simulink model "section4_simulation_editedbyzym"  (R2023b)
settings: Solver=FixedStepAuto  StartTime=0.0  StopTime=620  FixedStep=0.001  RelTol=1e-3
(part 2 of 2)

== matlab function section4_simulation_editedbyzym/droux ==
  data: krou input; y output; rou0 input; rou00 input; t input
function y = fcn(krou,rou0,rou00,t)
u=-krou*(rou0-rou00)*exp(-krou*t);
y = u;

== matlab function section4_simulation_editedbyzym/drouy1 ==
  data: krou input; y output; rou0 input; rou00 input; t input
function y = fcn(krou,rou0,rou00,t)
u=-krou*(rou0-rou00)*exp(-krou*t);
y = u;

== matlab function section4_simulation_editedbyzym/rouy1 ==
  data: rou0 input; y output; rou00 input; krou input; t input
function y = fcn(rou0,rou00,krou,t)
u=(rou0-rou00)*exp(-krou*t)+rou00;
y = u;

== matlab function section4_simulation_editedbyzym/MATLAB Function12 ==
  data: tauiL input; tauiR input; r input; J input; m input; dv1 output; domg1 output; l input
function [dv1,domg1] = fcn(tauiL,tauiR,r,J,m,l)

dv1=(tauiL+tauiR)/(m*r);

domg1=l*(tauiR-tauiL)/(J*r);

== matlab function section4_simulation_editedbyzym/MATLAB Function18 ==
  data: rphiL2 input; y output; thetaL input; theta2 input
function y = fcn(rphiL2,thetaL,theta2)
u=rphiL2+thetaL-theta2-pi/3;
y = u;

== matlab function section4_simulation_editedbyzym/MATLAB Function30 ==
  data: JIL output; JI1 output; JI2 output; JI3 output; x1 input; y1 input; x2 input; y2 input; x3 input; y3 input; xL input; yL input; yil output; sanyi output; yier output; saner output; erl output
function [JIL,JI1,JI2, JI3,yil,sanyi,yier,saner,erl]= fcn(x1,y1,x2,y2,x3,y3,xL,yL)
yil=sqrt((x1-xL)^2+(y1-yL)^2);
erl=sqrt((x2-xL)^2+(y2-yL)^2);
yier=sqrt((x2-x1)^2+(y2-y1)^2);
sanyi=sqrt((x3-x1)^2+(y3-y1)^2);
saner=sqrt((x3-x2)^2+(y3-y2)^2);
sanl=sqrt((x3-xL)^2+(y3-yL)^2);
JL=((yil)^2+(erl)^2-(yier)^2)/(2*yil*erl);
J1=((yil)^2+(sanyi)^2-(sanl)^2)/(2*yil*sanyi);
J2=((erl)^2+(saner)^2-(sanl)^2)/(2*erl*saner);
J3=((sanyi)^2+(saner)^2-(yier)^2)/(2*sanyi*saner);
JIL = acos(JL);
JI1 = acos(J1);
JI2 = acos(J2);
JI3 = acos(J3);

== matlab function section4_simulation_editedbyzym/phiL1 ==
  data: arfji output; xj input; phiji output; xi input; yj input; yi input; thetai input; thetaj input
function [arfji,phiji] = fcn(xj,xi,yj,yi,thetai,thetaj)
xji=cos(thetai)*(xj-xi)+sin(thetai)*(yj-yi);
yji=-sin(thetai)*(xj-xi)+cos(thetai)*(yj-yi);
arfji=atan(yji/xji);
phiji=arfji+thetai-thetaj;

== matlab function section4_simulation_editedbyzym/MATLAB Function1 ==
  data: aa input; tauiL output; bb input; cc input; dd input; uid input; uip input
function tauiL = fcn(aa,bb,cc,dd,uid,uip)

% if aa/bb-cc/dd<0.05 && aa/bb-cc/dd>-0.05
%     tauiL=1\(uid/bb-uip/dd);
% 
% 
% else 
tauiL=(aa/bb-cc/dd)\(uid/bb-uip/dd);
% end

== matlab function section4_simulation_editedbyzym/MATLAB Function2 ==
  data: aa input; tauiR output; bb input; cc input; dd input; uid input; uip input
function tauiR = fcn(aa,bb,cc,dd,uid,uip)

% if aa/bb-cc/dd<0.05 && aa/bb-cc/dd>-0.05
%     tauiR=1\(uid/aa-uip/cc);
% 
% else
tauiR=(bb/aa-dd/cc)\(uid/aa-uip/cc);
% end

== matlab function section4_simulation_editedbyzym/MATLAB Function9 ==
  data: gamma_id input; y output; sigma_id input; Didm_hat input; delta_id input
function y = fcn(gamma_id,sigma_id,Didm_hat,delta_id)


dot_Didm_hat=gamma_id*(abs(delta_id)-sigma_id*Didm_hat^3);

y = dot_Didm_hat;

== matlab function section4_simulation_editedbyzym/MATLAB Function33 ==
  data: gamma_id input; y output; sigma_id input; Didm_hat input; delta_id input
function y = fcn(gamma_id,sigma_id,Didm_hat,delta_id)


dot_Didm_hat=gamma_id*(abs(delta_id)-sigma_id*Didm_hat^3);

y = dot_Didm_hat;

== matlab function section4_simulation_editedbyzym/dot,dji1 ==
  data: vi input; y output; phiji input; h input; omgi input; omgj input; arfji input; vj input
function y = fcn(vi,phiji,h,omgi,omgj,arfji,vj)
u=-vi*cos(arfji)-h*omgi*sin(arfji)+vj*cos(phiji)+h*omgj*sin(phiji);
y = u;

== matlab function section4_simulation_editedbyzym/phiL2 ==
  data: arfji output; xj input; phiji output; xi input; yj input; yi input; thetai input; thetaj input
function [arfji,phiji] = fcn(xj,xi,yj,yi,thetai,thetaj)
xji=cos(thetai)*(xj-xi)+sin(thetai)*(yj-yi);
yji=-sin(thetai)*(xj-xi)+cos(thetai)*(yj-yi);
arfji=atan(yji/xji);
phiji=arfji+thetai-thetaj;

== matlab function section4_simulation_editedbyzym/dot,phiji1 ==
  data: omgi input; dphiji output; dji input; vi input; phiji input; h input; vj input; omgj input; darfji output; arfji input
function [dphiji,darfji] = fcn(omgi,dji,vi,phiji,h,vj,omgj,arfji)
dphiji=(dji)^(-1)*(-vj*sin(phiji)+h*omgj*cos(phiji)-h*omgi*cos(arfji)+vi*sin(arfji))-omgj;
darfji=(dji)^(-1)*(-dji*omgi-vj*sin(phiji)+h*omgj*cos(phiji)-h*omgi*cos(arfji)+vi*sin(arfji));

== matlab function section4_simulation_editedbyzym/MATLAB Function34 ==
  data: gamma_id input; y output; sigma_id input; Didm_hat input; delta_id input
function y = fcn(gamma_id,sigma_id,Didm_hat,delta_id)


dot_Didm_hat=gamma_id*(abs(delta_id)-sigma_id*Didm_hat^3);

y = dot_Didm_hat;

== matlab function section4_simulation_editedbyzym/MATLAB Function35 ==
  data: gamma_id input; y output; sigma_id input; Didm_hat input; delta_id input
function y = fcn(gamma_id,sigma_id,Didm_hat,delta_id)


dot_Didm_hat=gamma_id*(abs(delta_id)-sigma_id*Didm_hat^3);

y = dot_Didm_hat;

== matlab function section4_simulation_editedbyzym/MATLAB Function36 ==
  data: gamma_id input; y output; sigma_id input; Didm_hat input; delta_id input
function y = fcn(gamma_id,sigma_id,Didm_hat,delta_id)


dot_Didm_hat=gamma_id*(abs(delta_id)-sigma_id*Didm_hat^3);

y = dot_Didm_hat;

== matlab function section4_simulation_editedbyzym/u1p ==
  data: vj input; vi input; wj input; wi input; deltaip input; eip input; doteip input; roup input; dotroup input; ddotroup input; zip input; dotzip input; upzip input; lowzip input; phi input; dotphi input; y output; a input; dota input; kip input; h input; Dipm input; kiep input; d input; dotd input
function y = fcn(vj,vi,wj,wi,deltaip,eip,doteip,roup,dotroup,ddotroup,zip,dotzip,upzip,lowzip,phi,dotphi,a,dota,kip,h,Dipm,kiep,d,dotd)

if abs(deltaip)<0.1
u1=deltaip/0.1;
else
u1=sign(deltaip);
end

Cip=-vj*cos(phi)*dotphi-h*wj*sin(phi)*dotphi-wj*dotd-((doteip*dotroup*d+eip*ddotroup*d+eip*dotroup*dotd)*roup-eip*dotroup^2*d)/roup^2+kip*upzip^2*lowzip^2*((dotroup*zip*d+roup*dotzip*d+roup*zip*dotd)*(upzip-zip)*(zip+lowzip)-roup*zip*d*((-dotzip)*(zip+lowzip)+(dotzip)*(upzip-zip)))/((upzip-zip)^2*(zip+lowzip)^2);
Ciep=-h*wi*sin(a)*dota-vi*cos(a)*dota-(upzip^2*lowzip^2*(zip^2+upzip*lowzip)*zip)/((upzip-zip)^3*(zip+lowzip)^3*roup*d)-Cip;
uip=-Ciep-Dipm*u1-kiep*deltaip^3;

y = uip;

== matlab function section4_simulation_editedbyzym/MATLAB Function37 ==
  data: ks input; y output; t input
function y = fcn(ks,t)
if t>0&&t<=20
    u=0;
else
if t>20&&t<=320
  u=ks*(t-20);
  else
      u=ks*300;
end
end
y = u;

== matlab function section4_simulation_editedbyzym/a4 ==
  data: a input; y output; h input; l input; j input; r input; m input
function y = fcn(a,h,l,j,r,m)

u=cos(a)/(r*m)-h*l*sin(a)/(j*r);

y = u;

== matlab function section4_simulation_editedbyzym/a5 ==
  data: a input; y output; h input; l input; j input; r input; m input
function y = fcn(a,h,l,j,r,m)

u=cos(a)/(r*m)+h*l*sin(a)/(j*r);

y = u;

== matlab function section4_simulation_editedbyzym/MATLAB Function3 ==
  data: tauiL input; tauiR input; r input; J input; m input; dv1 output; domg1 output; l input
function [dv1,domg1] = fcn(tauiL,tauiR,r,J,m,l)

dv1=(tauiL+tauiR)/(m*r);

domg1=l*(tauiR-tauiL)/(J*r);

== matlab function section4_simulation_editedbyzym/MATLAB Function4 ==
  data: tauiL input; tauiR input; r input; J input; m input; dv1 output; domg1 output; l input
function [dv1,domg1] = fcn(tauiL,tauiR,r,J,m,l)

dv1=(tauiL+tauiR)/(m*r);

domg1=l*(tauiR-tauiL)/(J*r);

== matlab function section4_simulation_editedbyzym/MATLAB Function5 ==
  data: aa input; tauiL output; bb input; cc input; dd input; uid input; uip input
function tauiL = fcn(aa,bb,cc,dd,uid,uip)

% if aa/bb-cc/dd<0.05 && aa/bb-cc/dd>-0.05
%     tauiL=1\(uid/bb-uip/dd);
% 
% 
% else 
tauiL=(aa/bb-cc/dd)\(uid/bb-uip/dd);
% end

== matlab function section4_simulation_editedbyzym/MATLAB Function6 ==
  data: aa input; tauiR output; bb input; cc input; dd input; uid input; uip input
function tauiR = fcn(aa,bb,cc,dd,uid,uip)

% if aa/bb-cc/dd<0.05 && aa/bb-cc/dd>-0.05
%     tauiR=1\(uid/aa-uip/cc);
% 
% else
tauiR=(bb/aa-dd/cc)\(uid/aa-uip/cc);
% end

== matlab function section4_simulation_editedbyzym/d23 ==
  data: xi input; y output; xj input; yi input; yj input
function y = fcn(xi,xj,yi,yj)
u=sqrt((xj-xi)^2+(yj-yi)^2);
y = u;

== matlab function section4_simulation_editedbyzym/dot,dji2 ==
  data: vi input; y output; phiji input; h input; omgi input; omgj input; arfji input; vj input
function y = fcn(vi,phiji,h,omgi,omgj,arfji,vj)
u=-vi*cos(arfji)-h*omgi*sin(arfji)+vj*cos(phiji)+h*omgj*sin(phiji);
y = u;

== matlab function section4_simulation_editedbyzym/phi23 ==
  data: arfji output; xj input; phiji output; xi input; yj input; yi input; thetai input; thetaj input
function [arfji,phiji] = fcn(xj,xi,yj,yi,thetai,thetaj)
xji=cos(thetai)*(xj-xi)+sin(thetai)*(yj-yi);
yji=-sin(thetai)*(xj-xi)+cos(thetai)*(yj-yi);
arfji=atan(yji/xji);
phiji=arfji+thetai-thetaj;

== matlab function section4_simulation_editedbyzym/dot,phiji2 ==
  data: omgi input; dphiji output; dji input; vi input; phiji input; h input; vj input; omgj input; darfji output; arfji input
function [dphiji,darfji] = fcn(omgi,dji,vi,phiji,h,vj,omgj,arfji)
dphiji=(dji)^(-1)*(-vj*sin(phiji)+h*omgj*cos(phiji)-h*omgi*cos(arfji)+vi*sin(arfji))-omgj;
darfji=(dji)^(-1)*(-dji*omgi-vj*sin(phiji)+h*omgj*cos(phiji)-h*omgi*cos(arfji)+vi*sin(arfji));

== matlab function section4_simulation_editedbyzym/a6 ==
  data: a input; y output; h input; l input; j input; r input; m input
function y = fcn(a,h,l,j,r,m)

u=-sin(a)/(r*m)+h*l*cos(a)/(j*r);

y = u;

== matlab function section4_simulation_editedbyzym/u1d2 ==
  data: vj input; vi input; wj input; wi input; deltaid input; eid input; doteid input; roud input; dotroud input; ddotroud input; zid input; dotzid input; upzid input; lowzid input; phi input; dotphi input; y output; a input; dota input; kid input; h input; Didm input; kied input
function y = fcn(vj,vi,wj,wi,deltaid,eid,doteid,roud,dotroud,ddotroud,zid,dotzid,upzid,lowzid,phi,dotphi,a,dota,kid,h,Didm,kied)


if abs(deltaid)<0.1
u1=deltaid/0.1;
else
u1=sign(deltaid);
end

Cid=-vj*sin(phi)*dotphi+h*wj*cos(phi)*dotphi-((doteid*dotroud+eid*ddotroud)*roud-eid*dotroud^2)/roud^2+kid*upzid^2*lowzid^2*((dotroud*zid+roud*dotzid)*(upzid-zid)*(zid+lowzid)-roud*zid*((-dotzid)*(zid+lowzid)+(dotzid)*(upzid-zid)))/((upzid-zid)^2*(zid+lowzid)^2);
Cied=-vi*sin(a)*dota+h*wi*cos(a)*dota-(upzid^2*lowzid^2*(zid^2+upzid*lowzid)*zid)/((upzid-zid)^3*(zid+lowzid)^3*roud)-Cid;
uid=-Cied-Didm*u1-kied*deltaid^3;


y = uid;

== matlab function section4_simulation_editedbyzym/dL1 ==
  data: xi input; y output; xj input; yi input; yj input
function y = fcn(xi,xj,yi,yj)
u=sqrt((xj-xi)^2+(yj-yi)^2);
y = u;

== matlab function section4_simulation_editedbyzym/u1p2 ==
  data: vj input; vi input; wj input; wi input; deltaip input; eip input; doteip input; roup input; dotroup input; ddotroup input; zip input; dotzip input; upzip input; lowzip input; phi input; dotphi input; y output; a input; dota input; kip input; h input; Dipm input; kiep input; d input; dotd input
function y = fcn(vj,vi,wj,wi,deltaip,eip,doteip,roup,dotroup,ddotroup,zip,dotzip,upzip,lowzip,phi,dotphi,a,dota,kip,h,Dipm,kiep,d,dotd)

if abs(deltaip)<1
u1=deltaip/1;
else
u1=sign(deltaip);
end

Cip=-vj*cos(phi)*dotphi-h*wj*sin(phi)*dotphi-wj*dotd-((doteip*dotroup*d+eip*ddotroup*d+eip*dotroup*dotd)*roup-eip*dotroup^2*d)/roup^2+kip*upzip^2*lowzip^2*((dotroup*zip*d+roup*dotzip*d+roup*zip*dotd)*(upzip-zip)*(zip+lowzip)-roup*zip*d*((-dotzip)*(zip+lowzip)+(dotzip)*(upzip-zip)))/((upzip-zip)^2*(zip+lowzip)^2);
Ciep=-h*wi*sin(a)*dota-vi*cos(a)*dota-(upzip^2*lowzip^2*(zip^2+upzip*lowzip)*zip)/((upzip-zip)^3*(zip+lowzip)^3*roup*d)-Cip;
uip=-Ciep-Dipm*u1-kiep*deltaip^3;

y = uip;

== matlab function section4_simulation_editedbyzym/a7 ==
  data: a input; y output; h input; l input; j input; r input; m input
function y = fcn(a,h,l,j,r,m)

u=-sin(a)/(r*m)-h*l*cos(a)/(j*r);

y = u;

== matlab function section4_simulation_editedbyzym/a10 ==
  data: a input; y output; h input; l input; j input; r input; m input
function y = fcn(a,h,l,j,r,m)

u=-sin(a)/(r*m)+h*l*cos(a)/(j*r);

y = u;

== matlab function section4_simulation_editedbyzym/a11 ==
  data: a input; y output; h input; l input; j input; r input; m input
function y = fcn(a,h,l,j,r,m)

u=-sin(a)/(r*m)-h*l*cos(a)/(j*r);

y = u;

== matlab function section4_simulation_editedbyzym/a8 ==
  data: a input; y output; h input; l input; j input; r input; m input
function y = fcn(a,h,l,j,r,m)

u=cos(a)/(r*m)-h*l*sin(a)/(j*r);

y = u;

== matlab function section4_simulation_editedbyzym/MATLAB Function16 ==
  data: ks input; y output; t input
function y = fcn(ks,t)
if t>0&&t<=20
    u=0;
else
if t>20&&t<=320
  u=ks*(t-20);
  else
      u=ks*300;
end
end
y = u;

== matlab function section4_simulation_editedbyzym/a9 ==
  data: a input; y output; h input; l input; j input; r input; m input
function y = fcn(a,h,l,j,r,m)

u=cos(a)/(r*m)+h*l*sin(a)/(j*r);

y = u;

== matlab function section4_simulation_editedbyzym/MATLAB Function31 ==
  data: aa input; tauiL output; bb input; cc input; dd input; uid input; uip input
function tauiL = fcn(aa,bb,cc,dd,uid,uip)

% if aa/bb-cc/dd<0.05 && aa/bb-cc/dd>-0.05
%     tauiL=1\(uid/bb-uip/dd);
% 
% 
% else 
tauiL=(aa/bb-cc/dd)\(uid/bb-uip/dd);
% end

== matlab function section4_simulation_editedbyzym/MATLAB Function38 ==
  data: y output; t input
function y = fcn(t)
% if t>0&&t<5
%     u=0;
% else
%     if t>=5&&t<30
%        u=(t-5)*0.0016*pi/2;
%     else
%         if t>=30&&t<55
%             u = (55-t)*0.0016*pi/2;
%         else 
%             u=0;
%         end
%     end
% end
if t>0&&t<5
    u=0;
else
    if t>=5&&t<25
       u=-(t-5)*0.00260*pi/2;
    else
        if t>=25&&t<45
            u = -(45-t)*0.00260*pi/2;
        else 
            u=0;
        end
    end
end
% if t>0&&t<10
%     u=0;
% else
%     if t>=10&&t<30
%        u=(t-10)*0.00256*pi/2;
%     else
%         if t>=30&&t<50
%             u = (50-t)*0.00256*pi/2;
%         else 
%             u=0;
%         end
%     end
% end
y = u;

== matlab function section4_simulation_editedbyzym/MATLAB Function17 ==
  data: ks input; y output; t input
function y = fcn(ks,t)

u=0;

if t>0&&t<=20
    u=0;
elseif t>20&&t<=320
  u=ks*(t-20); 
elseif t>320
    u=ks*300-ks*(t-320);
end

y = u;

== matlab function section4_simulation_editedbyzym/MATLAB Function7 ==
  data: vj input; doted output; vi input; wj input; wi input; phi input; a input; h input
function doted = fcn(vj,vi,wj,wi,phi,a,h)

u=vj*cos(phi)+h*wj*sin(phi)-vi*cos(a)-h*wi*sin(a);

doted = u;

== matlab function section4_simulation_editedbyzym/MATLAB Function8 ==
  data: vj input; doted output; vi input; wj input; wi input; phi input; a input; h input
function doted = fcn(vj,vi,wj,wi,phi,a,h)

u=vj*cos(phi)+h*wj*sin(phi)-vi*cos(a)-h*wi*sin(a);

doted = u;

== matlab function section4_simulation_editedbyzym/MATLAB Function10 ==
  data: vj input; doted output; vi input; wj input; wi input; phi input; a input; h input
function doted = fcn(vj,vi,wj,wi,phi,a,h)

u=vj*cos(phi)+h*wj*sin(phi)-vi*cos(a)-h*wi*sin(a);

doted = u;

== matlab function section4_simulation_editedbyzym/MATLAB Function11 ==
  data: vj input; dotep output; vi input; wj input; wi input; phi input; a input; h input; d input
function dotep = fcn(vj,vi,wj,wi,phi,a,h,d)

u=(-vj*sin(phi)+h*wj*cos(phi)-h*wi*cos(a)+vi*sin(a))/d-wj;

dotep = u;

== matlab function section4_simulation_editedbyzym/MATLAB Function13 ==
  data: vj input; dotep output; vi input; wj input; wi input; phi input; a input; h input; d input
function dotep = fcn(vj,vi,wj,wi,phi,a,h,d)

u=(-vj*sin(phi)+h*wj*cos(phi)-h*wi*cos(a)+vi*sin(a))/d-wj;

dotep = u;

== matlab function section4_simulation_editedbyzym/MATLAB Function14 ==
  data: vj input; dotep output; vi input; wj input; wi input; phi input; a input; h input; d input
function dotep = fcn(vj,vi,wj,wi,phi,a,h,d)

u=(-vj*sin(phi)+h*wj*cos(phi)-h*wi*cos(a)+vi*sin(a))/d-wj;

dotep = u;

== matlab function section4_simulation_editedbyzym/ddroux2 ==
  data: krou input; y output; rou0 input; rou00 input; t input
function y = fcn(krou,rou0,rou00,t)
u=krou*krou*(rou0-rou00)*exp(-krou*t);
y = u;

== matlab function section4_simulation_editedbyzym/u1d ==
  data: vj input; vi input; wj input; wi input; deltaid input; eid input; doteid input; roud input; dotroud input; ddotroud input; zid input; dotzid input; upzid input; lowzid input; phi input; dotphi input; y output; a input; dota input; kid input; h input; Didm input; kied input
function y = fcn(vj,vi,wj,wi,deltaid,eid,doteid,roud,dotroud,ddotroud,zid,dotzid,upzid,lowzid,phi,dotphi,a,dota,kid,h,Didm,kied)


if abs(deltaid)<0.1
u1=deltaid/0.1;
else
u1=sign(deltaid);
end

Cid=-vj*sin(phi)*dotphi+h*wj*cos(phi)*dotphi-((doteid*dotroud+eid*ddotroud)*roud-eid*dotroud^2)/roud^2+kid*upzid^2*lowzid^2*((dotroud*zid+roud*dotzid)*(upzid-zid)*(zid+lowzid)-roud*zid*((-dotzid)*(zid+lowzid)+(dotzid)*(upzid-zid)))/((upzid-zid)^2*(zid+lowzid)^2);
Cied=-vi*sin(a)*dota+h*wi*cos(a)*dota-(upzid^2*lowzid^2*(zid^2+upzid*lowzid)*zid)/((upzid-zid)^3*(zid+lowzid)^3*roud)-Cid;
uid=-Cied-Didm*u1-kied*deltaid^3;


y = uid;

== matlab function section4_simulation_editedbyzym/dL2 ==
  data: xi input; y output; xj input; yi input; yj input
function y = fcn(xi,xj,yi,yj)
u=sqrt((xj-xi)^2+(yj-yi)^2);
y = u;

== matlab function section4_simulation_editedbyzym/ddrouy ==
  data: krou input; y output; rou0 input; rou00 input; t input
function y = fcn(krou,rou0,rou00,t)
u=krou*krou*(rou0-rou00)*exp(-krou*t);
y = u;

== matlab function section4_simulation_editedbyzym/MATLAB Function15 ==
  data: vj input; delta1 output; vi input; wj input; wi input; a input; phi input; h input; ed input; roud input; droud input; zd input; upzd input; lowzd input; kd input
function delta1 = fcn(vj,vi,wj,wi,a,phi,h,ed,roud,droud,zd,upzd,lowzd,kd)
u1=vi*cos(a)+h*wi*sin(a);
u1d=vj*cos(phi)+h*wj*sin(phi)-(ed*droud)/roud+kd*(upzd^2*lowzd^2*roud*zd)/((upzd-roud)*(roud+lowzd));
delta1 = u1-u1d;

== matlab function section4_simulation_editedbyzym/MATLAB Function19 ==
  data: vj input; delta2 output; vi input; wj input; wi input; a input; phi input; h input; ep input; roup input; droup input; zp input; upzp input; lowzp input; kp input; d input
function delta2 = fcn(vj,vi,wj,wi,a,phi,h,ep,roup,droup,zp,upzp,lowzp,kp,d)
u2=h*wi*cos(a)-vi*sin(a);
u2d=-vj*sin(phi)+h*wj*cos(phi)-wj*d-(ep*droup*d)/roup+kp*(upzp^2*lowzp^2*roup*zp*d)/((upzp-roup)*(roup+lowzp));
delta2 = u2-u2d;

== matlab function section4_simulation_editedbyzym/MATLAB Function20 ==
  data: vj input; delta1 output; vi input; wj input; wi input; a input; phi input; h input; ed input; roud input; droud input; zd input; upzd input; lowzd input; kd input
function delta1 = fcn(vj,vi,wj,wi,a,phi,h,ed,roud,droud,zd,upzd,lowzd,kd)
u1=vi*cos(a)+h*wi*sin(a);
u1d=vj*cos(phi)+h*wj*sin(phi)-(ed*droud)/roud+kd*(upzd^2*lowzd^2*roud*zd)/((upzd-roud)*(roud+lowzd));
delta1 = u1-u1d;

== matlab function section4_simulation_editedbyzym/MATLAB Function21 ==
  data: vj input; delta2 output; vi input; wj input; wi input; a input; phi input; h input; ep input; roup input; droup input; zp input; upzp input; lowzp input; kp input; d input
function delta2 = fcn(vj,vi,wj,wi,a,phi,h,ep,roup,droup,zp,upzp,lowzp,kp,d)
u2=h*wi*cos(a)-vi*sin(a);
u2d=-vj*sin(phi)+h*wj*cos(phi)-wj*d-(ep*droup*d)/roup+kp*(upzp^2*lowzp^2*roup*zp*d)/((upzp-roup)*(roup+lowzp));
delta2 = u2-u2d;

== matlab function section4_simulation_editedbyzym/dot,dji ==
  data: vi input; y output; phiji input; h input; omgi input; omgj input; arfji input; vj input
function y = fcn(vi,phiji,h,omgi,omgj,arfji,vj)
u=-vi*cos(arfji)-h*omgi*sin(arfji)+vj*cos(phiji)+h*omgj*sin(phiji);
y = u;

== matlab function section4_simulation_editedbyzym/MATLAB Function22 ==
  data: vj input; delta1 output; vi input; wj input; wi input; a input; phi input; h input; ed input; roud input; droud input; zd input; upzd input; lowzd input; kd input
function delta1 = fcn(vj,vi,wj,wi,a,phi,h,ed,roud,droud,zd,upzd,lowzd,kd)
u1=vi*cos(a)+h*wi*sin(a);
u1d=vj*cos(phi)+h*wj*sin(phi)-(ed*droud)/roud+kd*(upzd^2*lowzd^2*roud*zd)/((upzd-roud)*(roud+lowzd));
delta1 = u1-u1d;

== matlab function section4_simulation_editedbyzym/MATLAB Function23 ==
  data: vj input; delta2 output; vi input; wj input; wi input; a input; phi input; h input; ep input; roup input; droup input; zp input; upzp input; lowzp input; kp input; d input
function delta2 = fcn(vj,vi,wj,wi,a,phi,h,ep,roup,droup,zp,upzp,lowzp,kp,d)
u2=h*wi*cos(a)-vi*sin(a);
u2d=-vj*sin(phi)+h*wj*cos(phi)-wj*d-(ep*droup*d)/roup+kp*(upzp^2*lowzp^2*roup*zp*d)/((upzp-roup)*(roup+lowzp));
delta2 = u2-u2d;

== matlab function section4_simulation_editedbyzym/MATLAB Function24 ==
  data: eid input; y output; doteid input; roud input; dotroud input
function y = fcn(eid,doteid,roud,dotroud)

u=(doteid*roud-eid*dotroud)/roud^2;

y = u;

== matlab function section4_simulation_editedbyzym/MATLAB Function25 ==
  data: eid input; y output; doteid input; roud input; dotroud input
function y = fcn(eid,doteid,roud,dotroud)

u=(doteid*roud-eid*dotroud)/roud^2;

y = u;

== matlab function section4_simulation_editedbyzym/MATLAB Function26 ==
  data: eid input; y output; doteid input; roud input; dotroud input
function y = fcn(eid,doteid,roud,dotroud)

u=(doteid*roud-eid*dotroud)/roud^2;

y = u;

== matlab function section4_simulation_editedbyzym/MATLAB Function27 ==
  data: eip input; y output; doteip input; roup input; dotroup input
function y = fcn(eip,doteip,roup,dotroup)

u=(doteip*roup-eip*dotroup)/roup^2;

y = u;

== matlab function section4_simulation_editedbyzym/MATLAB Function28 ==
  data: eip input; y output; doteip input; roup input; dotroup input
function y = fcn(eip,doteip,roup,dotroup)

u=(doteip*roup-eip*dotroup)/roup^2;

y = u;

== matlab function section4_simulation_editedbyzym/MATLAB Function29 ==
  data: eip input; y output; doteip input; roup input; dotroup input
function y = fcn(eip,doteip,roup,dotroup)

u=(doteip*roup-eip*dotroup)/roup^2;

y = u;

== matlab function section4_simulation_editedbyzym/a ==
  data: a input; y output; h input; l input; j input; r input; m input
function y = fcn(a,h,l,j,r,m)

u=cos(a)/(r*m)-h*l*sin(a)/(j*r);

y = u;

== matlab function section4_simulation_editedbyzym/a1 ==
  data: a input; y output; h input; l input; j input; r input; m input
function y = fcn(a,h,l,j,r,m)

u=cos(a)/(r*m)+h*l*sin(a)/(j*r);

y = u;

== matlab function section4_simulation_editedbyzym/MATLAB Function ==
  data: gamma_id input; y output; sigma_id input; Didm_hat input; delta_id input
function y = fcn(gamma_id,sigma_id,Didm_hat,delta_id)


dot_Didm_hat=gamma_id*(abs(delta_id)-sigma_id*Didm_hat^3);

y = dot_Didm_hat;

== matlab function section4_simulation_editedbyzym/a2 ==
  data: a input; y output; h input; l input; j input; r input; m input
function y = fcn(a,h,l,j,r,m)

u=-sin(a)/(r*m)+h*l*cos(a)/(j*r);

y = u;

== matlab function section4_simulation_editedbyzym/a3 ==
  data: a input; y output; h input; l input; j input; r input; m input
function y = fcn(a,h,l,j,r,m)

u=-sin(a)/(r*m)-h*l*cos(a)/(j*r);

y = u;

== matlab function section4_simulation_editedbyzym/MATLAB Function32 ==
  data: aa input; tauiR output; bb input; cc input; dd input; uid input; uip input
function tauiR = fcn(aa,bb,cc,dd,uid,uip)

% if aa/bb-cc/dd<0.05 && aa/bb-cc/dd>-0.05
%     tauiR=1\(uid/aa-uip/cc);
% 
% else
tauiR=(bb/aa-dd/cc)\(uid/aa-uip/cc);
% end

== matlab function section4_simulation_editedbyzym/alpha1 ==
  data: y output; t input
function y = fcn(t)
if t>0&&t<=20
    u=0;%%初始跑一段直线
else
if t>20&&t<=(77.6)
  u=3.1545*10^(-4)*(t-20);%%从直线进入回旋线
else
    if t>77.6&&t<135.2
       u=3.1545*10^(-4)*135.2-3.1545*10^(-4)*(t);%%omgL=0，出回旋线准备画圆
    else 
        if t>=135.2&&t<=140
            u=0; %%  跑一小段直线，以便取个整数时间点
        else
            if t>140&&t<=150
                u=-1.5*10^(-3)*(t-140);%%进入回旋线(omgL逐渐增大)准备跑圆
            else
                if t>150&&t<=310
                u=-1.5*10^(-3)*10;%%跑圆
                else
                    if t>310&&t<=357.5
                    u=-1.5*10^(-3)*10+3.1545*10^(-4)*(t-310);%%出回旋线(omgL归零)，准备以更大角速度转向
                    else
                        if t>357.5&&t<=362
                        u=-3*10^(-3)*(t-357.5);%%进回旋线(omgL重新增加),准备以更快的角速度转弯
                        else
                            if t>362&&t<=520
                            u=-3*10^(-3)*(362-357.5);%%保持该角速度画圆，并取个整数时间点
                            else
                                if t>520&&t<=580
                                u=-3*10^(-3)*(362-357.5)-3.1545*10^(-4)*(t-520);%%出回旋线(omgL减小)，
                                else
                                    if t>580&&t<=600
                                    u=-3*10^(-3)*(362-357.5)-3.1545*10^(-4)*(580-520)+1*10^(-3)*(t-580);%%进入新的回旋线以获得更大的角加速度进行转弯
                                    else
                                        if t>600&&t<=680
                                        u=-3*10^(-3)*(362-357.5)-3.1545*10^(-4)*(580-520)+1*10^(-3)*(600-580);%%保持较大的角速度进行画圆
                                         %u=-0.0124;
                                        else
                                        u=-0.0124+4.15*10^(-4)*(t-680);%%出回旋线(减小omgL)，结束画圆并收尾
                                        end
                                    end
                                end
                            end
                        end
                    end
                end
                
            end
        end
                
    end
end
end
y = u;

== matlab function section4_simulation_editedbyzym/u1d1 ==
  data: vj input; vi input; wj input; wi input; deltaid input; eid input; doteid input; roud input; dotroud input; ddotroud input; zid input; dotzid input; upzid input; lowzid input; phi input; dotphi input; y output; a input; dota input; kid input; h input; Didm input; kied input
function y = fcn(vj,vi,wj,wi,deltaid,eid,doteid,roud,dotroud,ddotroud,zid,dotzid,upzid,lowzid,phi,dotphi,a,dota,kid,h,Didm,kied)


if abs(deltaid)<0.1
u1=deltaid/0.1;
else
u1=sign(deltaid);
end

Cid=-vj*sin(phi)*dotphi+h*wj*cos(phi)*dotphi-((doteid*dotroud+eid*ddotroud)*roud-eid*dotroud^2)/roud^2+kid*upzid^2*lowzid^2*((dotroud*zid+roud*dotzid)*(upzid-zid)*(zid+lowzid)-roud*zid*((-dotzid)*(zid+lowzid)+(dotzid)*(upzid-zid)))/((upzid-zid)^2*(zid+lowzid)^2);
Cied=-vi*sin(a)*dota+h*wi*cos(a)*dota-(upzid^2*lowzid^2*(zid^2+upzid*lowzid)*zid)/((upzid-zid)^3*(zid+lowzid)^3*roud)-Cid;
uid=-Cied-Didm*u1-kied*deltaid^3;


y = uid;

== matlab function section4_simulation_editedbyzym/u1p1 ==
  data: vj input; vi input; wj input; wi input; deltaip input; eip input; doteip input; roup input; dotroup input; ddotroup input; zip input; dotzip input; upzip input; lowzip input; phi input; dotphi input; y output; a input; dota input; kip input; h input; Dipm input; kiep input; d input; dotd input
function y = fcn(vj,vi,wj,wi,deltaip,eip,doteip,roup,dotroup,ddotroup,zip,dotzip,upzip,lowzip,phi,dotphi,a,dota,kip,h,Dipm,kiep,d,dotd)

if abs(deltaip)<0.1
u1=deltaip/0.1;
else
u1=sign(deltaip);
end

Cip=-vj*cos(phi)*dotphi-h*wj*sin(phi)*dotphi-wj*dotd-((doteip*dotroup*d+eip*ddotroup*d+eip*dotroup*dotd)*roup-eip*dotroup^2*d)/roup^2+kip*upzip^2*lowzip^2*((dotroup*zip*d+roup*dotzip*d+roup*zip*dotd)*(upzip-zip)*(zip+lowzip)-roup*zip*d*((-dotzip)*(zip+lowzip)+(dotzip)*(upzip-zip)))/((upzip-zip)^2*(zip+lowzip)^2);
Ciep=-h*wi*sin(a)*dota-vi*cos(a)*dota-(upzip^2*lowzip^2*(zip^2+upzip*lowzip)*zip)/((upzip-zip)^3*(zip+lowzip)^3*roup*d)-Cip;
uip=-Ciep-Dipm*u1-kiep*deltaip^3;

y = uip;

== matlab function section4_simulation_editedbyzym/dot,phiji ==
  data: omgi input; dphiji output; dji input; vi input; phiji input; h input; vj input; omgj input; darfji output; arfji input
function [dphiji,darfji] = fcn(omgi,dji,vi,phiji,h,vj,omgj,arfji)
dphiji=(dji)^(-1)*(-vj*sin(phiji)+h*omgj*cos(phiji)-h*omgi*cos(arfji)+vi*sin(arfji))-omgj;
darfji=(dji)^(-1)*(-dji*omgi-vj*sin(phiji)+h*omgj*cos(phiji)-h*omgi*cos(arfji)+vi*sin(arfji));

== matlab function section4_simulation_editedbyzym/roux1 ==
  data: rou0 input; y output; rou00 input; krou input; t input
function y = fcn(rou0,rou00,krou,t)
u=(rou0-rou00)*exp(-krou*t)+rou00;
y = u;
